simulink library "tetherBuoyancyAndWeightNGreater2_ul"  (R2018b)
settings: Solver=VariableStepAuto  StartTime=0.0  StopTime=10.0  RelTol=1e-3
values from neighbouring files (symbols this model uses):
  N = 4    [tetherBuoyAndWeight_ts.m]
  rho_fluid = 1000    [tetherBuoyAndWeight_ts.m]
  rho_tether = 1010    [tetherBuoyAndWeight_ts.m]
libraries: simulink x1, cylinderVolume_ul x1
settings Model: Creator=asiddiq2  LastModifiedBy=asiddiq2

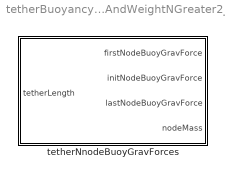
== system tetherBuoyancyAndWeightNGreater2_ul ==
  tetherNnodeBuoyGravForces : Subsystem  mask{rhoFluid=rho_fluid, gravAccl=10, numNode=4, diaTether=1, rhoTether=rho_tether}
      mask prompts: rhoFluid "Fluid density"; gravAccl "Gravitational acceleration"; numNode "Number of nodes"; diaTether "Tether diameter"; rhoTether "Tether density"
      mask DialogControl Container3 Prompt: Environment

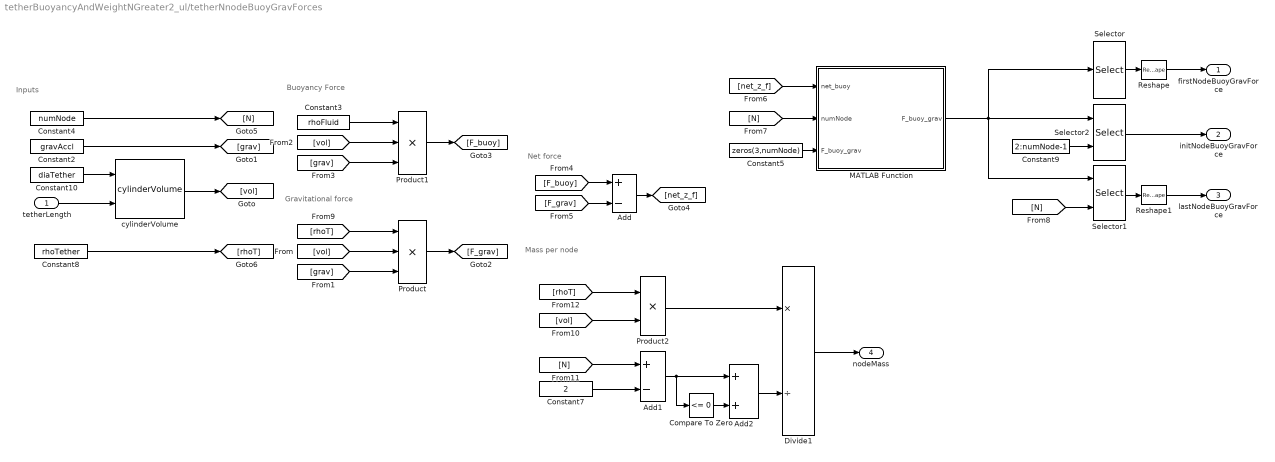
== system tetherBuoyancyAndWeightNGreater2_ul/tetherNnodeBuoyGravForces ==
  note: Inputs
  note: Mass per node
  note: Net force
  note: Buoyancy Force
  note: Gravitational force
  tetherLength : Inport
  Add : Sum  Inputs=+-
  Add1 : Sum  Inputs=+-
  Add2 : Sum
  Compare To Zero : simulink/Logic and Bit Operations/Compare To Zero  relop=<=  OutDataTypeStr=boolean
  Constant10 : Constant  Value=diaTether  VectorParams1D=off
  Constant2 : Constant  Value=gravAccl  VectorParams1D=off
  Constant3 : Constant  Value=rhoFluid  VectorParams1D=off
  Constant4 : Constant  Value=numNode  VectorParams1D=off
  Constant5 : Constant  Value=zeros(3,numNode)  VectorParams1D=off
  Constant7 : Constant  Value=2
  Constant8 : Constant  Value=rhoTether  VectorParams1D=off
  Constant9 : Constant  Value=2:numNode-1  VectorParams1D=off
  Divide1 : Product  Inputs=*/
  MATLAB Function : MATLAB Function  TreatAsAtomicUnit=on
  Product : Product  Inputs=3
  Product1 : Product  Inputs=3
  Product2 : Product
  Reshape : Reshape  OutputDimensionality=Column vector (2-D)
  Reshape1 : Reshape  OutputDimensionality=Column vector (2-D)
  Selector : Selector  NumberOfDimensions=2  InputPortWidth=3  IndexOptions=Select all,Index vector (dialog)  Indices=[1 3],1  OutputSizes=1,1
  Selector1 : Selector  NumberOfDimensions=2  InputPortWidth=3  IndexOptions=Select all,Index vector (port)  Indices=[1 3],N  OutputSizes=1,1
  Selector2 : Selector  NumberOfDimensions=2  InputPortWidth=3  IndexOptions=Select all,Index vector (port)  Indices=[1 3],[2:N-1]  OutputSizes=1,1
  cylinderVolume : cylinderVolume_ul/cylinderVolume  SystemSampleTime=-1
  firstNodeBuoyGravForce : Outport
  initNodeBuoyGravForce : Outport  Port=2
  lastNodeBuoyGravForce : Outport  Port=3
  nodeMass : Outport  Port=4
  wires:
  tetherLength/1 -> cylinderVolume/2
  cylinderVolume/1 -> [vol]
  Constant2/1 -> [grav]
  [rhoT] -> Product/1
  [vol] -> Product/2
  [grav] -> Product/3
  Product/1 -> [F_grav]
  [grav] -> Product1/3
  Constant3/1 -> Product1/1
  [vol] -> Product1/2
  Product1/1 -> [F_buoy]
  [F_buoy] -> Add/1
  [F_grav] -> Add/2
  Add/1 -> [net_z_f]
  [net_z_f] -> MATLAB Function/1(net_buoy)
  Constant4/1 -> [N]
  [N] -> MATLAB Function/2(numNode)
  Constant5/1 -> MATLAB Function/3("F_buoy_grav ")
  [vol] -> Product2/2
  [rhoT] -> Product2/1
  Product2/1 -> Divide1/1
  Divide1/1 -> nodeMass/1
  [N] -> Add1/1
  Add1/1 -> Compare To Zero/1, Add2/1
  Constant7/1 -> Add1/2
  Compare To Zero/1 -> Add2/2
  Add2/1 -> Divide1/2
  [N] -> Selector1/2
  MATLAB Function/1(F_buoy_grav) -> Selector1/1, Selector/1, Selector2/1
  Selector2/1 -> initNodeBuoyGravForce/1
  Selector/1 -> Reshape/1
  Selector1/1 -> Reshape1/1
  Constant9/1 -> Selector2/2
  Reshape/1 -> firstNodeBuoyGravForce/1
  Reshape1/1 -> lastNodeBuoyGravForce/1
  Constant10/1 -> cylinderVolume/1
  Constant8/1 -> [rhoT]

== matlab function tetherBuoyancyAndWeightNGreater2_ul/tetherNnodeBuoyGravForces/MATLAB Function ==
  data: net_buoy input; F_buoy_grav output; numNode input; F_buoy_grav input
function F_buoy_grav = fcn(net_buoy,numNode,F_buoy_grav)

for i = 1:numNode
    if i == 1
        F_buoy_grav(:,i) = zeros(3,1);
    elseif i>1 && i<numNode
        F_buoy_grav(:,i) = net_buoy/(numNode-2)*[0; 0; 1];
    elseif i == numNode
        F_buoy_grav(:,i) = zeros(3,1);
    end
    
end

end
